simulink model "park"  (R2023a)
settings: Solver=VariableStepAuto  StartTime=0.0  StopTime=10.0  RelTol=1e-3
values from neighbouring files (symbols this model uses):
  k = 1    [park_init.m]
undefined symbols (not defined in the file or in its folder): DiscIntNeverNeededParam
settings Model: Creator=11048  LastModifiedBy=11048

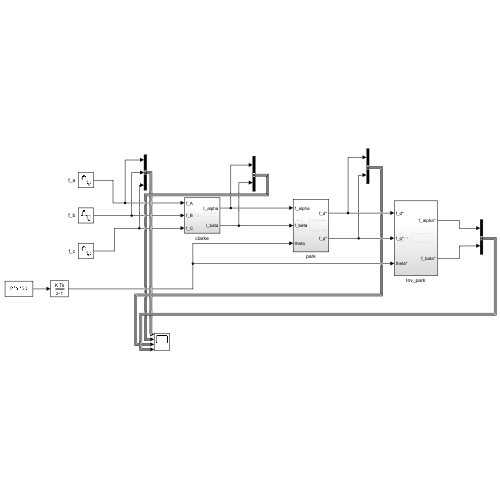
[thumbnail: Simulink's stored preview of the top-level diagram]
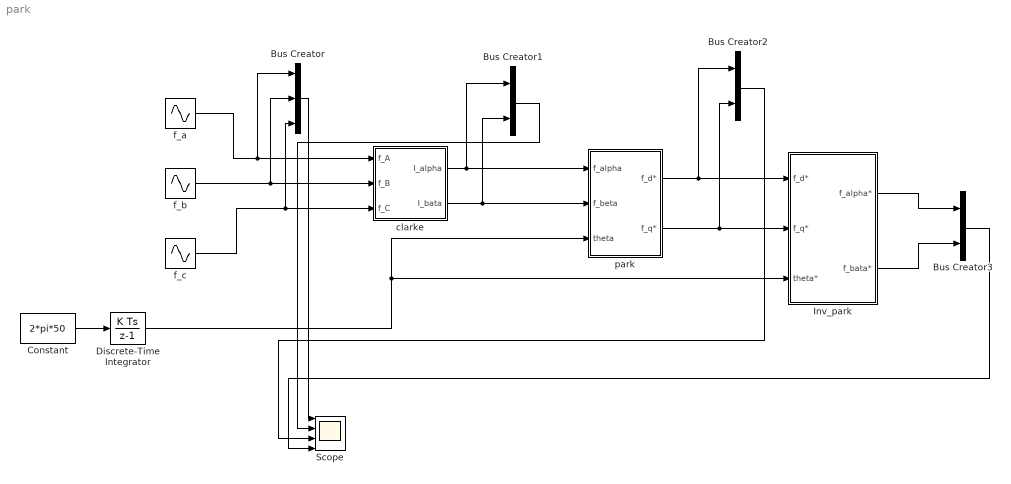
== system park ==
  Bus Creator : BusCreator  Inputs=3
  Bus Creator1 : BusCreator  Inputs=2
  Bus Creator2 : BusCreator  Inputs=2
  Bus Creator3 : BusCreator  Inputs=2
  Constant : Constant  Value=2*pi*50
  Discrete-Time Integrator : DiscreteIntegrator  SampleTime=-1  ICPrevOutput=DiscIntNeverNeededParam  ICPrevScaledInput=DiscIntNeverNeededParam
  Inv_park : Subsystem
  Scope : Scope  NumInputPorts=4
  clarke : Subsystem
  f_a : Sin  Frequency=2*pi*50  SampleTime=0.00001
  f_b : Sin  Frequency=2*pi*50  Phase=-pi*2/3  SampleTime=0.00001
  f_c : Sin  Frequency=2*pi*50  Phase=pi*2/3  SampleTime=0.00001
  park : Subsystem
  wires:
  clarke/1(I_alpha) -> Bus Creator1/1, park/1(f_alpha)
  clarke/2(I_bata) -> Bus Creator1/2, park/2(f_beta)
  f_a/1 -> Bus Creator/1, clarke/1(f_A)
  f_b/1 -> Bus Creator/2, clarke/2(f_B)
  f_c/1 -> Bus Creator/3, clarke/3(f_C)
  park/1(f_d*) -> Bus Creator2/1, Inv_park/1(f_d*)
  park/2(f_q*) -> Bus Creator2/2, Inv_park/2(f_q*)
  Discrete-Time Integrator/1 -> Inv_park/3(theta*), park/3(theta)
  Inv_park/1(f_alpha*) -> Bus Creator3/1
  Inv_park/2(f_bata*) -> Bus Creator3/2
  Bus Creator2/1 -> Scope/3
  Bus Creator/1 -> Scope/1
  Bus Creator1/1 -> Scope/2
  Bus Creator3/1 -> Scope/4
  Constant/1 -> Discrete-Time Integrator/1

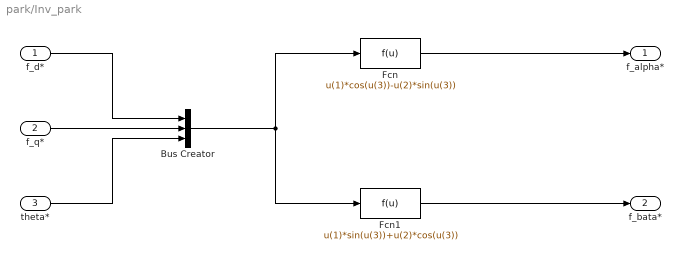
== system park/Inv_park ==
  f_d* : Inport
  f_q* : Inport  Port=2
  theta* : Inport  Port=3
  Bus Creator : BusCreator  Inputs=3
  Fcn : Fcn  Expr=u(1)*cos(u(3))-u(2)*sin(u(3))
  Fcn1 : Fcn  Expr=u(1)*sin(u(3))+u(2)*cos(u(3))
  f_alpha* : Outport
  f_bata* : Outport  Port=2
  wires:
  Fcn1/1 -> f_bata*/1
  f_q*/1 -> Bus Creator/2
  Fcn/1 -> f_alpha*/1
  Bus Creator/1 -> Fcn1/1, Fcn/1
  theta*/1 -> Bus Creator/3
  f_d*/1 -> Bus Creator/1

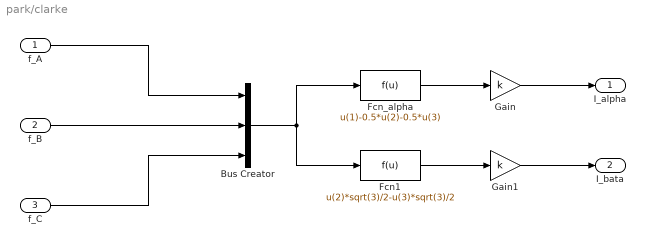
== system park/clarke ==
  f_A : Inport
  f_B : Inport  Port=2
  f_C : Inport  Port=3
  Bus Creator : BusCreator  Inputs=3
  Fcn1 : Fcn  Expr=u(2)*sqrt(3)/2-u(3)*sqrt(3)/2
  Fcn_alpha : Fcn  Expr=u(1)-0.5*u(2)-0.5*u(3)
  Gain : Gain  Gain=k
  Gain1 : Gain  Gain=k
  I_alpha : Outport
  I_bata : Outport  Port=2
  wires:
  Bus Creator/1 -> Fcn1/1, Fcn_alpha/1
  f_A/1 -> Bus Creator/1
  f_C/1 -> Bus Creator/3
  f_B/1 -> Bus Creator/2
  Fcn_alpha/1 -> Gain/1
  Gain/1 -> I_alpha/1
  Fcn1/1 -> Gain1/1
  Gain1/1 -> I_bata/1

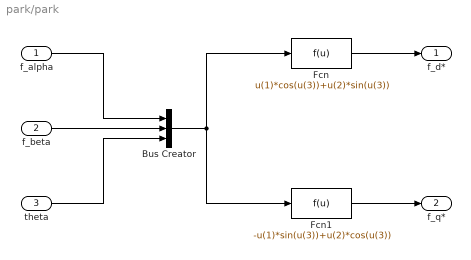
== system park/park ==
  f_alpha : Inport
  f_beta : Inport  Port=2
  theta : Inport  Port=3
  Bus Creator : BusCreator  Inputs=3
  Fcn : Fcn  Expr=u(1)*cos(u(3))+u(2)*sin(u(3))
  Fcn1 : Fcn  Expr=-u(1)*sin(u(3))+u(2)*cos(u(3))
  f_d* : Outport
  f_q* : Outport  Port=2
  wires:
  f_beta/1 -> Bus Creator/2
  Bus Creator/1 -> Fcn1/1, Fcn/1
  f_alpha/1 -> Bus Creator/1
  theta/1 -> Bus Creator/3
  Fcn1/1 -> f_q*/1
  Fcn/1 -> f_d*/1
